simulink model "Lift_off_state"  (R2017b)
settings: Solver=VariableStepAuto  StartTime=0.0  StopTime=10.0  RelTol=1e-3
settings Model: Creator=Kalana  LastModifiedBy=Kalana

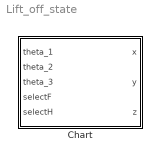
== system Lift_off_state ==
  Chart : Stateflow chart  TreatAsAtomicUnit=on

== stateflow chart Lift_off_state/Chart ==
  state Set_State_Swing
    entry: x = -0.310*sin(theta_1)*cos(theta_2-theta_3)-0.255*sin(theta_1)*cos(theta_2)-0.14*sin(theta_1);
    y = -0.310*sin(theta_2-theta_3)-0.255*sin(theta_2);
    z = -0.310*cos(theta_1)*cos(theta_2-theta_3)-0.255*cos(theta_1)*cos(theta_2)-0.14*cos(theta_1);
  state Fixed_State_State
    entry: x = x
    y = y
    z = z
  (default) -> Set_State_Swing
  Set_State_Swing -> Fixed_State_State : [selectF*selectH==1 ]
  Fixed_State_State -> Set_State_Swing : [selectF+selectH == 0]
  data: theta_1 input; theta_2 input; theta_3 input; x output; y output; z output; selectF input; selectH input
